simulink model "model"  (R2022a)
settings: Solver=VariableStepAuto  StartTime=0.0  StopTime=Inf  RelTol=1e-3
settings Model: Creator=mateu  LastModifiedBy=mateu

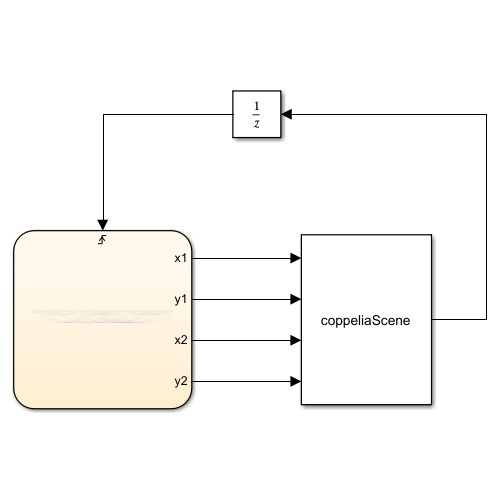
[thumbnail: Simulink's stored preview of the top-level diagram]
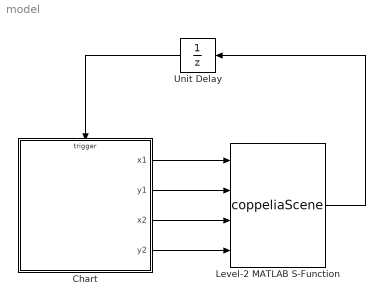
== system model ==
  Chart : Stateflow chart  TreatAsAtomicUnit=on
  Level-2 MATLAB S-Function : M-S-Function  FunctionName=coppeliaScene
  Unit Delay : UnitDelay  SampleTime=-1  HasFrameUpgradeWarning=on
  wires:
  Chart/1(x1) -> Level-2 MATLAB S-Function/1
  Chart/2(y1) -> Level-2 MATLAB S-Function/2
  Chart/3(x2) -> Level-2 MATLAB S-Function/3
  Chart/4(y2) -> Level-2 MATLAB S-Function/4
  Unit Delay/1 -> Chart/Trigger
  Level-2 MATLAB S-Function/1 -> Unit Delay/1

== stateflow chart model/Chart ==
  settings: executeAtInitialization=1
  state parallel_plant_sup
    state s01
      x1=1;
      y1=1;
      x2=1;
      y2=2;
    state s02
      x1=1;
      y1=1;
      x2=1;
      y2=3;
    state s03
      x1=1;
      y1=1;
      x2=2;
      y2=1;
    state s04
      x1=1;
      y1=1;
      x2=2;
      y2=2;
    state s05
      x1=1;
      y1=1;
      x2=2;
      y2=3;
    state s06
      x1=1;
      y1=1;
      x2=3;
      y2=1;
    state s07
      x1=1;
      y1=1;
      x2=3;
      y2=2;
    state s08
      x1=1;
      y1=1;
      x2=3;
      y2=3;
    state s09
      x1=1;
      y1=2;
      x2=1;
      y2=1;
    state s010
      x1=1;
      y1=2;
      x2=2;
      y2=1;
    state s011
      x1=1;
      y1=2;
      x2=2;
      y2=2;
    state s012
      x1=1;
      y1=2;
      x2=2;
      y2=3;
    state s013
      x1=1;
      y1=2;
      x2=3;
      y2=1;
    state s014
      x1=1;
      y1=2;
      x2=3;
      y2=2;
    state s015
      x1=1;
      y1=2;
      x2=3;
      y2=3;
    state s016
      x1=1;
      y1=3;
      x2=1;
      y2=1;
    state s017
      x1=1;
      y1=3;
      x2=1;
      y2=2;
    state s018
      x1=1;
      y1=3;
      x2=2;
      y2=1;
    state s019
      x1=1;
      y1=3;
      x2=2;
      y2=2;
    state s020
      x1=1;
      y1=3;
      x2=2;
      y2=3;
    state s021
      x1=1;
      y1=3;
      x2=3;
      y2=1;
    state s022
      x1=1;
      y1=3;
      x2=3;
      y2=2;
    state s023
      x1=1;
      y1=3;
      x2=3;
      y2=3;
    state s024
      x1=2;
      y1=1;
      x2=1;
      y2=1;
    state s025
      x1=2;
      y1=1;
      x2=1;
      y2=2;
    state s026
      x1=2;
      y1=1;
      x2=1;
      y2=3;
    state s027
      x1=2;
      y1=1;
      x2=2;
      y2=2;
    state s028
      x1=2;
      y1=1;
      x2=2;
      y2=3;
    state s029
      x1=2;
      y1=1;
      x2=3;
      y2=1;
    state s030
      x1=2;
      y1=1;
      x2=3;
      y2=2;
    state s031
      x1=2;
      y1=1;
      x2=3;
      y2=3;
    state s032
      x1=2;
      y1=2;
      x2=1;
      y2=1;
    state s033
      x1=2;
      y1=2;
      x2=1;
      y2=2;
    state s034
      x1=2;
      y1=2;
      x2=1;
      y2=3;
    state s035
      x1=2;
      y1=2;
      x2=2;
      y2=1;
    state s036
      x1=2;
      y1=2;
      x2=2;
      y2=3;
    state s037
      x1=2;
      y1=2;
      x2=3;
      y2=1;
    state s038
      x1=2;
      y1=2;
      x2=3;
      y2=3;
    state s039
      x1=2;
      y1=3;
      x2=1;
      y2=1;
    state s040
      x1=2;
      y1=3;
      x2=1;
      y2=2;
    state s041
      x1=2;
      y1=3;
      x2=1;
      y2=3;
    state s042
      x1=2;
      y1=3;
      x2=2;
      y2=1;
    state s043
      x1=2;
      y1=3;
      x2=2;
      y2=2;
    state s044
      x1=2;
      y1=3;
      x2=3;
      y2=1;
    state s045
      x1=2;
      y1=3;
      x2=3;
      y2=2;
    state s046
      x1=2;
      y1=3;
      x2=3;
      y2=3;
    state s047
      x1=3;
      y1=1;
      x2=1;
      y2=1;
    state s048
      x1=3;
      y1=1;
      x2=1;
      y2=2;
    state s049
      x1=3;
      y1=1;
      x2=1;
      y2=3;
    state s050
      x1=3;
      y1=1;
      x2=2;
      y2=1;
    state s051
      x1=3;
      y1=1;
      x2=2;
      y2=2;
    state s052
      x1=3;
      y1=1;
      x2=2;
      y2=3;
    state s053
      x1=3;
      y1=1;
      x2=3;
      y2=2;
    state s054
      x1=3;
      y1=1;
      x2=3;
      y2=3;
    state s055
      x1=3;
      y1=2;
      x2=1;
      y2=1;
    state s056
      x1=3;
      y1=2;
      x2=1;
      y2=2;
    state s057
      x1=3;
      y1=2;
      x2=1;
      y2=3;
    state s058
      x1=3;
      y1=2;
      x2=2;
      y2=1;
    state s059
      x1=3;
      y1=2;
      x2=2;
      y2=2;
    state s060
      x1=3;
      y1=2;
      x2=2;
      y2=3;
    state s061
      x1=3;
      y1=2;
      x2=3;
      y2=1;
    state s062
      x1=3;
      y1=2;
      x2=3;
      y2=3;
    state s063
      x1=3;
      y1=3;
      x2=1;
      y2=1;
    state s064
      x1=3;
      y1=3;
      x2=1;
      y2=2;
    state s065
      x1=3;
      y1=3;
      x2=1;
      y2=3;
    state s066
      x1=3;
      y1=3;
      x2=2;
      y2=1;
    state s067
      x1=3;
      y1=3;
      x2=2;
      y2=2;
    state s068
      x1=3;
      y1=3;
      x2=2;
      y2=3;
    state s069
      x1=3;
      y1=3;
      x2=3;
      y2=1;
    state s070
      x1=3;
      y1=3;
      x2=3;
      y2=2;
    (default) -> s06
    s02 -> s01 [order 2] : R2d
    s02 -> s01 [order 4] : R2ureq
    s04 -> s01 [order 4] : R2l
    s025 -> s01 [order 1] : R1l
    s01 -> s025 [order 1] : R1r
    s01 -> s04 [order 2] : R2r
    s01 -> s02 [order 3] : R2u
    s05 -> s02 [order 4] : R2l
    s026 -> s02 [order 1] : R1l
    s02 -> s026 [order 1] : R1r
    s02 -> s05 [order 3] : R2r
    s04 -> s03 [order 3] : R2d
    s06 -> s03 [order 3] : R2l
    s010 -> s03 [order 1] : R1d
    s03 -> s010 [order 1] : R1u
    s03 -> s06 [order 2] : R2r
    s03 -> s04 [order 3] : R2u
    s05 -> s04 [order 3] : R2d
    s07 -> s04 [order 4] : R2l
    s011 -> s04 [order 1] : R1d
    s027 -> s04 [order 1] : R1l
    s04 -> s027 [order 1] : R1r
    s04 -> s011 [order 2] : R1u
    s04 -> s07 [order 5] : R2r
    s04 -> s05 [order 6] : R2u
    s08 -> s05 [order 4] : R2l
    s012 -> s05 [order 1] : R1d
    s028 -> s05 [order 1] : R1l
    s05 -> s028 [order 1] : R1r
    s05 -> s012 [order 2] : R1u
    s05 -> s08 [order 5] : R2r
    s07 -> s06 [order 3] : R2d
    s013 -> s06 [order 1] : R1d
    s029 -> s06 [order 1] : R1l
    s06 -> s029 [order 1] : R1r
    s06 -> s013 [order 2] : R1u
    s06 -> s07 [order 4] : R2u
    s08 -> s07 [order 3] : R2d
    s014 -> s07 [order 1] : R1d
    s030 -> s07 [order 1] : R1l
    s07 -> s030 [order 1] : R1r
    s07 -> s014 [order 2] : R1u
    s07 -> s08 [order 5] : R2u
    s015 -> s08 [order 1] : R1d
    s031 -> s08 [order 1] : R1l
    s08 -> s031 [order 1] : R1r
    s08 -> s015 [order 2] : R1u
    s010 -> s09 [order 4] : R2l
    s016 -> s09 [order 1] : R1d
    s032 -> s09 [order 2] : R1l
    s09 -> s032 [order 1] : R1r
    s09 -> s016 [order 2] : R1u
    s09 -> s010 [order 3] : R2r
    s011 -> s010 [order 3] : R2d
    s013 -> s010 [order 4] : R2l
    s018 -> s010 [order 1] : R1d
    s035 -> s010 [order 1] : R1l
    s010 -> s035 [order 2] : R1r
    s010 -> s018 [order 3] : R1u
    s010 -> s013 [order 5] : R2r
    s010 -> s011 [order 6] : R2u
    s012 -> s011 [order 4] : R2d
    s014 -> s011 [order 4] : R2l
    s019 -> s011 [order 1] : R1d
    s011 -> s019 [order 2] : R1u
    s011 -> s014 [order 4] : R2r
    s011 -> s012 [order 5] : R2u
    s015 -> s012 [order 5] : R2l
    s020 -> s012 [order 1] : R1d
    s036 -> s012 [order 2] : R1l
    s012 -> s036 [order 2] : R1r
    s012 -> s020 [order 3] : R1u
    s012 -> s015 [order 5] : R2r
    s014 -> s013 [order 3] : R2d
    s021 -> s013 [order 1] : R1d
    s037 -> s013 [order 2] : R1l
    s013 -> s037 [order 2] : R1r
    s013 -> s021 [order 3] : R1u
    s013 -> s014 [order 5] : R2u
    s015 -> s014 [order 4] : R2d
    s022 -> s014 [order 1] : R1d
    s014 -> s022 [order 2] : R1u
    s014 -> s015 [order 5] : R2u
    s023 -> s015 [order 1] : R1d
    s038 -> s015 [order 2] : R1l
    s015 -> s038 [order 2] : R1r
    s015 -> s023 [order 3] : R1u
    s017 -> s016 [order 2] : R2d
    s018 -> s016 [order 3] : R2l
    s039 -> s016 [order 2] : R1l
    s016 -> s039 [order 2] : R1r
    s016 -> s018 [order 3] : R2r
    s016 -> s017 [order 4] : R2u
    s019 -> s017 [order 4] : R2l
    s040 -> s017 [order 2] : R1l
    s017 -> s040 [order 1] : R1r
    s017 -> s019 [order 3] : R2r
    s019 -> s018 [order 3] : R2d
    s021 -> s018 [order 3] : R2l
    s042 -> s018 [order 2] : R1l
    s018 -> s042 [order 2] : R1r
    s018 -> s021 [order 4] : R2r
    s018 -> s019 [order 5] : R2u
    s020 -> s019 [order 2] : R2d
    s022 -> s019 [order 4] : R2l
    s043 -> s019 [order 1] : R1l
    s019 -> s043 [order 2] : R1r
    s019 -> s022 [order 5] : R2r
    s019 -> s020 [order 6] : R2u
    s023 -> s020 [order 4] : R2l
    s020 -> s023 [order 3] : R2r
    s022 -> s021 [order 3] : R2d
    s044 -> s021 [order 2] : R1l
    s021 -> s044 [order 2] : R1r
    s021 -> s022 [order 4] : R2u
    s023 -> s022 [order 3] : R2d
    s045 -> s022 [order 1] : R1l
    s022 -> s045 [order 2] : R1r
    s022 -> s023 [order 5] : R2u
    s046 -> s023 [order 2] : R1l
    s023 -> s046 [order 2] : R1r
    s025 -> s024 [order 4] : R2d
    s032 -> s024 [order 1] : R1d
    s047 -> s024 [order 1] : R1l
    s024 -> s047 [order 1] : R1r
    s024 -> s032 [order 2] : R1u
    s024 -> s025 [order 3] : R2u
    s026 -> s025 [order 4] : R2d
    s026 -> s025 [order 6] : R2ureq
    s027 -> s025 [order 3] : R2l
    s033 -> s025 [order 1] : R1d
    s048 -> s025 [order 1] : R1l
    s025 -> s048 [order 2] : R1r
    s025 -> s033 [order 3] : R1u
    s025 -> s027 [order 5] : R2r
    s025 -> s026 [order 6] : R2u
    s028 -> s026 [order 5] : R2l
    s034 -> s026 [order 1] : R1d
    s049 -> s026 [order 1] : R1l
    s026 -> s049 [order 2] : R1r
    s026 -> s034 [order 3] : R1u
    s026 -> s028 [order 5] : R2r
    s028 -> s027 [order 4] : R2d
    s030 -> s027 [order 4] : R2l
    s051 -> s027 [order 1] : R1l
    s027 -> s051 [order 2] : R1r
    s027 -> s030 [order 4] : R2r
    s027 -> s028 [order 5] : R2u
    s031 -> s028 [order 5] : R2l
    s036 -> s028 [order 1] : R1d
    s052 -> s028 [order 1] : R1l
    s028 -> s052 [order 2] : R1r
    s028 -> s036 [order 3] : R1u
    s028 -> s031 [order 6] : R2r
    s030 -> s029 [order 3] : R2d
    s037 -> s029 [order 1] : R1d
    s029 -> s037 [order 2] : R1u
    s029 -> s030 [order 3] : R2u
    s031 -> s030 [order 4] : R2d
    s053 -> s030 [order 1] : R1l
    s030 -> s053 [order 2] : R1r
    s030 -> s031 [order 5] : R2u
    s038 -> s031 [order 1] : R1d
    s054 -> s031 [order 1] : R1l
    s031 -> s054 [order 2] : R1r
    s031 -> s038 [order 3] : R1u
    s033 -> s032 [order 5] : R2d
    s035 -> s032 [order 5] : R2l
    s039 -> s032 [order 1] : R1d
    s055 -> s032 [order 2] : R1l
    s032 -> s055 [order 3] : R1r
    s032 -> s039 [order 4] : R1u
    s032 -> s055 [order 5] : R1ureq
    s032 -> s035 [order 6] : R2r
    s032 -> s033 [order 7] : R2u
    s034 -> s033 [order 5] : R2d
    s034 -> s033 [order 7] : R2ureq
    s040 -> s033 [order 1] : R1d
    s056 -> s033 [order 2] : R1l
    s033 -> s056 [order 2] : R1r
    s033 -> s040 [order 3] : R1u
    s033 -> s056 [order 4] : R1ureq
    s033 -> s034 [order 6] : R2u
    s036 -> s034 [order 5] : R2l
    s041 -> s034 [order 1] : R1d
    s057 -> s034 [order 2] : R1l
    s034 -> s057 [order 2] : R1r
    s034 -> s041 [order 3] : R1u
    s034 -> s057 [order 4] : R1ureq
    s034 -> s036 [order 6] : R2r
    s037 -> s035 [order 6] : R2l
    s042 -> s035 [order 1] : R1d
    s058 -> s035 [order 2] : R1l
    s035 -> s058 [order 2] : R1r
    s035 -> s042 [order 3] : R1u
    s035 -> s058 [order 4] : R1ureq
    s035 -> s037 [order 6] : R2r
    s038 -> s036 [order 6] : R2l
    s060 -> s036 [order 2] : R1l
    s036 -> s060 [order 3] : R1r
    s036 -> s060 [order 4] : R1ureq
    s036 -> s038 [order 6] : R2r
    s044 -> s037 [order 1] : R1d
    s061 -> s037 [order 1] : R1l
    s037 -> s061 [order 3] : R1r
    s037 -> s044 [order 4] : R1u
    s037 -> s061 [order 5] : R1ureq
    s046 -> s038 [order 1] : R1d
    s062 -> s038 [order 2] : R1l
    s038 -> s062 [order 3] : R1r
    s038 -> s046 [order 4] : R1u
    s038 -> s062 [order 5] : R1ureq
    s040 -> s039 [order 4] : R2d
    s042 -> s039 [order 4] : R2l
    s063 -> s039 [order 2] : R1l
    s039 -> s063 [order 3] : R1r
    s039 -> s042 [order 4] : R2r
    s039 -> s040 [order 5] : R2u
    s041 -> s040 [order 3] : R2d
    s041 -> s040 [order 4] : R2ureq
    s043 -> s040 [order 4] : R2l
    s064 -> s040 [order 2] : R1l
    s040 -> s064 [order 3] : R1r
    s040 -> s043 [order 5] : R2r
    s040 -> s041 [order 6] : R2u
    s065 -> s041 [order 2] : R1l
    s041 -> s065 [order 2] : R1r
    s043 -> s042 [order 3] : R2d
    s044 -> s042 [order 4] : R2l
    s066 -> s042 [order 2] : R1l
    s042 -> s066 [order 3] : R1r
    s042 -> s044 [order 5] : R2r
    s042 -> s043 [order 6] : R2u
    s045 -> s043 [order 4] : R2l
    s067 -> s043 [order 2] : R1l
    s043 -> s067 [order 2] : R1r
    s043 -> s045 [order 5] : R2r
    s045 -> s044 [order 3] : R2d
    s069 -> s044 [order 2] : R1l
    s044 -> s069 [order 3] : R1r
    s044 -> s045 [order 5] : R2u
    s046 -> s045 [order 3] : R2d
    s070 -> s045 [order 1] : R1l
    s045 -> s070 [order 2] : R1r
    s045 -> s046 [order 5] : R2u
    s048 -> s047 [order 3] : R2d
    s050 -> s047 [order 2] : R2l
    s055 -> s047 [order 1] : R1d
    s047 -> s055 [order 2] : R1u
    s047 -> s050 [order 3] : R2r
    s047 -> s048 [order 4] : R2u
    s049 -> s048 [order 3] : R2d
    s049 -> s048 [order 5] : R2ureq
    s051 -> s048 [order 4] : R2l
    s056 -> s048 [order 1] : R1d
    s048 -> s056 [order 2] : R1u
    s048 -> s051 [order 4] : R2r
    s048 -> s049 [order 5] : R2u
    s052 -> s049 [order 4] : R2l
    s057 -> s049 [order 1] : R1d
    s049 -> s057 [order 2] : R1u
    s049 -> s052 [order 4] : R2r
    s051 -> s050 [order 3] : R2d
    s058 -> s050 [order 1] : R1d
    s050 -> s058 [order 1] : R1u
    s050 -> s051 [order 3] : R2u
    s052 -> s051 [order 3] : R2d
    s053 -> s051 [order 2] : R2l
    s059 -> s051 [order 1] : R1d
    s051 -> s059 [order 2] : R1u
    s051 -> s053 [order 5] : R2r
    s051 -> s052 [order 6] : R2u
    s054 -> s052 [order 4] : R2l
    s060 -> s052 [order 1] : R1d
    s052 -> s060 [order 2] : R1u
    s052 -> s054 [order 5] : R2r
    s054 -> s053 [order 3] : R2d
    s053 -> s054 [order 3] : R2u
    s062 -> s054 [order 1] : R1d
    s054 -> s062 [order 2] : R1u
    s056 -> s055 [order 4] : R2d
    s058 -> s055 [order 4] : R2l
    s063 -> s055 [order 1] : R1d
    s055 -> s063 [order 3] : R1u
    s055 -> s058 [order 4] : R2r
    s055 -> s056 [order 5] : R2u
    s057 -> s056 [order 4] : R2d
    s057 -> s056 [order 6] : R2ureq
    s059 -> s056 [order 4] : R2l
    s064 -> s056 [order 1] : R1d
    s056 -> s064 [order 3] : R1u
    s056 -> s059 [order 5] : R2r
    s056 -> s057 [order 6] : R2u
    s060 -> s057 [order 5] : R2l
    s065 -> s057 [order 1] : R1d
    s057 -> s065 [order 3] : R1u
    s057 -> s060 [order 5] : R2r
    s059 -> s058 [order 3] : R2d
    s061 -> s058 [order 3] : R2l
    s066 -> s058 [order 1] : R1d
    s058 -> s066 [order 3] : R1u
    s058 -> s061 [order 5] : R2r
    s058 -> s059 [order 6] : R2u
    s060 -> s059 [order 4] : R2d
    s067 -> s059 [order 1] : R1d
    s059 -> s067 [order 2] : R1u
    s059 -> s060 [order 5] : R2u
    s062 -> s060 [order 3] : R2l
    s068 -> s060 [order 1] : R1d
    s060 -> s068 [order 3] : R1u
    s060 -> s062 [order 6] : R2r
    s069 -> s061 [order 1] : R1d
    s061 -> s069 [order 2] : R1u
    s064 -> s063 [order 3] : R2d
    s066 -> s063 [order 3] : R2l
    s063 -> s066 [order 3] : R2r
    s063 -> s064 [order 4] : R2u
    s065 -> s064 [order 3] : R2d
    s065 -> s064 [order 5] : R2ureq
    s067 -> s064 [order 4] : R2l
    s064 -> s067 [order 4] : R2r
    s064 -> s065 [order 5] : R2u
    s068 -> s065 [order 3] : R2l
    s065 -> s068 [order 4] : R2r
    s067 -> s066 [order 3] : R2d
    s069 -> s066 [order 3] : R2l
    s066 -> s069 [order 4] : R2r
    s066 -> s067 [order 5] : R2u
    s068 -> s067 [order 2] : R2d
    s070 -> s067 [order 3] : R2l
    s067 -> s070 [order 5] : R2r
    s067 -> s068 [order 6] : R2u
    s070 -> s069 [order 2] : R2d
    s069 -> s070 [order 4] : R2u
  (default) -> parallel_plant_sup
  data: x1 output; y1 output; x2 output; y2 output
  events: R1d input RISING_EDGE_EVENT; R1l input RISING_EDGE_EVENT; R1r input RISING_EDGE_EVENT; R1u input RISING_EDGE_EVENT; R1ureq input RISING_EDGE_EVENT; R2d input RISING_EDGE_EVENT; R2l input RISING_EDGE_EVENT; R2r input RISING_EDGE_EVENT; R2u input RISING_EDGE_EVENT; R2ureq input RISING_EDGE_EVENT
